simulink model "rover_dual_control"  (R2024b)
settings: Solver=FixedStepDiscrete  StartTime=0.0  StopTime=inf  FixedStep=0.1  RelTol=1e-3
InitFcn:
  | dualRoot = fileparts(fileparts(get_param(bdroot, 'FileName'))); addpath(fullfile(dualRoot, 'matlab')); addpath(fullfile(fileparts(dualRoot), 'matlab')); addpath(fullfile(fileparts(dualRoot), 'roversim', 'MATLAB')); rover_dual_init();
StartFcn:
  | dualRoot = fileparts(fileparts(get_param(bdroot, 'FileName'))); addpath(fullfile(dualRoot, 'matlab')); addpath(fullfile(fileparts(dualRoot), 'matlab')); addpath(fullfile(fileparts(dualRoot), 'roversim', 'MATLAB')); rover_dual_start();
StopFcn:
  | dualRoot = fileparts(fileparts(get_param(bdroot, 'FileName'))); addpath(fullfile(dualRoot, 'matlab')); addpath(fullfile(fileparts(dualRoot), 'matlab')); addpath(fullfile(fileparts(dualRoot), 'roversim', 'MATLAB')); rover_dual_stop();
undefined symbols (not defined in the file): angular, linear, simulink_map_pose_to_unreal, simulink_mcl_map_pose, simulink_teleop_ang, simulink_teleop_lin, simulink_unreal_pose_gate
libraries: sim3dlib x3, ros2lib x2
settings Model: Creator=dinuk  LastModifiedBy=dinuk

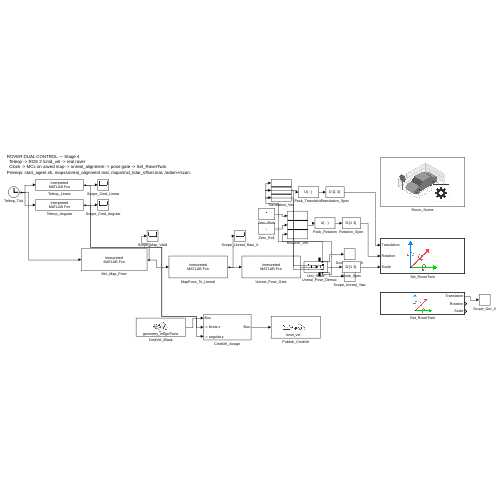
[thumbnail: Simulink's stored preview of the top-level diagram]
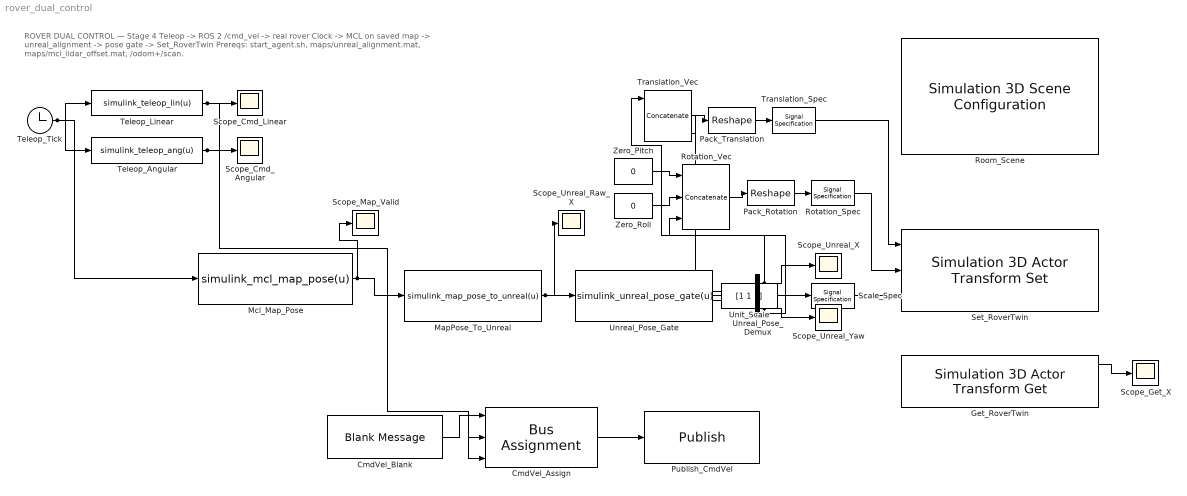
== system rover_dual_control ==
  note: ROVER DUAL CONTROL — Stage 4
      |   Teleop -> ROS 2 /cmd_vel -> real rover
      |   Clock -> MCL on saved map -> unreal_alignment -> pose gate -> Set_RoverTwin
      | Prereqs: start_agent.sh, maps/unreal_alignment.mat, maps/mcl_lidar_offset.mat, /odom+/scan.
  CmdVel_Assign : BusAssignment  AssignedSignals=linear.x,angular.z
  CmdVel_Blank : ros2lib/Blank Message  messageClass=Message  entityType=geometry_msgs/Twist  messageType=geometry_msgs/Twist  SampleTime=0
      link override Constant: OutDataTypeStr=Bus: SL_Bus_geometry_msgs_Twist
  Get_RoverTwin : sim3dlib/Simulation 3D Actor Transform Get  Priority=1  ActorTag=RoverTwin  NumberOfParts=1  CustNumOfParts=3  Ts=-1  aMode=aMode
  MapPose_To_Unreal : MATLABFcn  MATLABFcn=simulink_map_pose_to_unreal(u)  OutputDimensions=4
  Mcl_Map_Pose : MATLABFcn  MATLABFcn=simulink_mcl_map_pose(u)  OutputDimensions=4
  Pack_Rotation : Reshape  OutputDimensions=[1 3]
  Pack_Translation : Reshape  OutputDimensions=[1 3]
  Publish_CmdVel : ros2lib/Publish  topicSource=Specify your own  topic=/cmd_vel  messageType=geometry_msgs/Twist  QOSHistory=Keep last  QOSDepth=10  QOSReliability=Reliable  QOSDurability=Volatile  QOSDeadline=Inf  QOSLifespan=Inf  QOSLiveliness=Automatic  QOSLeaseDuration=Inf  QOSAvoidROSNamespaceConventions=off
      link override SinkBlock: ROSTopic=/cmd_vel  ROSMessageType=geometry_msgs/Twist  SLBusName=SL_Bus_geometry_msgs_Twist  ModelName=rover_dual_control  BlockId=Pub_rover_dual_control_30
  Room_Scene : sim3dlib/Simulation 3D Scene Configuration  Priority=0  ProjectFormat=Unreal Editor  SceneDesc=Straight road  ProjectName=/home/dinuk/MATLAB/R2024b/toolbox/shared/sim3d_projects/automotive_project_linux/UE/LinuxNoEditor/VehicleSimulation.sh  ScenePath=/Game/Maps/MyRoom  UEProjPath=/tmp/RoverTwinUnrealProject/RoverTwin/RoverTwin.uproject  EnableOpenDRIVE=off  vehTagList="{\"Scene Origin\", \"RoverTwin\"}"  vehTag=RoverTwin  FreeCameraInitialTranslation=[2.9725352 1.565026 1.03]  FreeCameraDefaultInitialTranslation=[-6, 0, 2]  FreeCameraInitialRotation=[-15, 0, 0]  FreeCameraDefaultInitialRotation=[0, -15, 0]  OpVisEn=off  Ts=0.1  EnableWindow=on  EnableRemoteAccess=off  EnableWeather=off  SunAzimuth=90  SunAltitude=40.0  EnableGeospatialSun=off  Latitude=0  Longitude=0  Date=2023-01-01  Time=10:30:00  GeoTimeZone=-5.0  SunDaylightSaving=off  wind=1  clouds=10  EnableVolumetricClouds=off  CloudCoverage=0  CloudAltitude=6  fog=0  rain=0  RaindropsEffect=off  SnowDensity=0  EnableGeospatial=off  UseTrueOrigin=off  OriginHeight=200  OriginLatitude=40.744652  OriginLongitude=-73.988864  MapStyle=Aerial  AdditionalAssetIDs=[]  UseAdvancedSunSky=off  SolarTime=11  TimeZone=-5  Day=21  Month=9  Year=2022  UseDaylightSavingTime=on  DSTStartDay=10  DSTStartMonth=3  DSTEndDay=3  DSTEndMonth=11  DSTSwitchHour=2  sensorTag=MainCamera1  sensorId=1  sensorName=MainCamera1  mountLoc=Origin  offsetFlag=off  tmountOffset=[0, 0, 0]  rmountOffset=[0, 0, 0]  HorizontalResolution=1280  VerticalResolution=720  HorizontalFOV=60  mountPoint=[0 0 0]  mountOrientation=[0 0 0]  aMode=3  ID=1  GeoTrigger=Inactive
      settings: LibrarySourceBlock=drivingsim3d/Simulation 3D Scene Configuration
  Rotation_Spec : SignalSpecification  Dimensions=[1 3]
  Rotation_Vec : Concatenate  NumInputs=3  ConcatenateDimension=2
  Scale_Spec : SignalSpecification  Dimensions=[1 3]
  Scope_Cmd_Angular : Scope
  Scope_Cmd_Linear : Scope
  Scope_Get_X : Scope
  Scope_Map_Valid : Scope
  Scope_Unreal_Raw_X : Scope
  Scope_Unreal_X : Scope
  Scope_Unreal_Yaw : Scope
  Set_RoverTwin : sim3dlib/Simulation 3D Actor Transform Set  Priority=-2  ActorTag=RoverTwin  NumberOfParts=1  CustNumOfParts=3  Translation=[1.25 0.8 -1.47]  Rotation=[0 0 0]  Scale=[1 1 1]  Ts=0.1  aMode=aMode
  Teleop_Angular : MATLABFcn  MATLABFcn=simulink_teleop_ang(u)
  Teleop_Linear : MATLABFcn  MATLABFcn=simulink_teleop_lin(u)
  Teleop_Tick : Clock
  Translation_Spec : SignalSpecification  Dimensions=[1 3]
  Translation_Vec : Concatenate  NumInputs=3  ConcatenateDimension=2
  Unit_Scale : Constant  Value=[1 1 1]  VectorParams1D=off
  Unreal_Pose_Demux : Demux
  Unreal_Pose_Gate : MATLABFcn  MATLABFcn=simulink_unreal_pose_gate(u)  OutputDimensions=4
  Zero_Pitch : Constant  Value=0
  Zero_Roll : Constant  Value=0
  wires:
  Teleop_Tick/1 -> Teleop_Linear/1, Teleop_Angular/1, Mcl_Map_Pose/1
  Teleop_Linear/1 -> Scope_Cmd_Linear/1, CmdVel_Assign/2
  Teleop_Angular/1 -> Scope_Cmd_Angular/1, CmdVel_Assign/3
  Mcl_Map_Pose/1 -> MapPose_To_Unreal/1, Scope_Map_Valid/1
  MapPose_To_Unreal/1 -> Unreal_Pose_Gate/1, Scope_Unreal_Raw_X/1
  Unreal_Pose_Gate/1 -> Unreal_Pose_Demux/1
  Unreal_Pose_Demux/1 -> Scope_Unreal_X/1, Translation_Vec/1
  Unreal_Pose_Demux/4 -> Scope_Unreal_Yaw/1, Rotation_Vec/3
  Translation_Vec/1 -> Pack_Translation/1
  Pack_Translation/1 -> Translation_Spec/1
  Rotation_Vec/1 -> Pack_Rotation/1
  Pack_Rotation/1 -> Rotation_Spec/1
  Unreal_Pose_Demux/2 -> Translation_Vec/2
  Unreal_Pose_Demux/3 -> Translation_Vec/3
  Zero_Pitch/1 -> Rotation_Vec/1
  Zero_Roll/1 -> Rotation_Vec/2
  Unit_Scale/1 -> Scale_Spec/1
  Translation_Spec/1 -> Set_RoverTwin/1
  Rotation_Spec/1 -> Set_RoverTwin/2
  Scale_Spec/1 -> Set_RoverTwin/3
  Get_RoverTwin/1 -> Scope_Get_X/1
  CmdVel_Blank/1 -> CmdVel_Assign/1
  CmdVel_Assign/1 -> Publish_CmdVel/1
